simulink model "halfCar"  (R2017b)
settings: Solver=ode23t  StartTime=0.0  StopTime=10  FixedStep=0.05  RelTol=1e-3
settings Model: Creator=cs756  LastModifiedBy=cs756

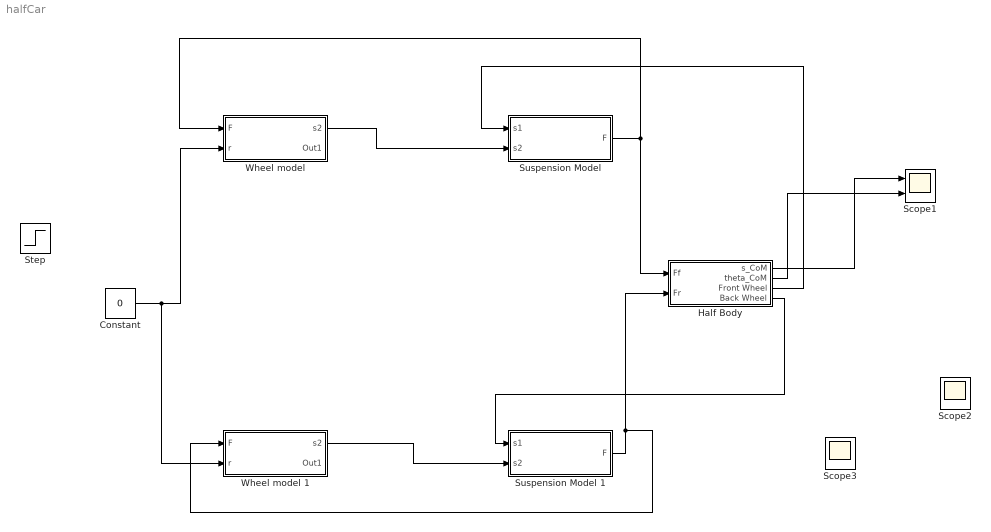
== system halfCar ==
  Constant : Constant  Value=0
  Half Body : Subsystem  mask{g=9.81, I=600, mb=500, a=1.25, b=1.4}
  Scope1 : Scope  NumInputPorts=2
  Scope2 : Scope
  Scope3 : Scope
  Step : Step  SampleTime=0
  "Suspension Model " : Subsystem  mask{cs1=1000, cs2=1000, ks=20000, ks2=20000, x0=2, x1=2}
      mask prompts: cs1 "Damper Compression coefficient"; cs2 "Damper Tension coefficient"; ks "Stiffness coefficient"; ks2 "Stiffness addition"; x0 "Elastic spring extension limit"; x1 "Damper motion range"
  Suspension Model 1 : Subsystem  mask{cs1=1000, cs2=1000, ks=20000, ks2=20000, x0=2, x1=2}
      mask prompts: cs1 "Damper Compression coefficient"; cs2 "Damper Tension coefficient"; ks "Stiffness coefficient"; ks2 "Stiffness addition"; x0 "Elastic spring extension limit"; x1 "Damper motion range"
  "Wheel model " : Subsystem  mask{kt=140000, kt2=140000, m2=20, g=9.81, x0=1}
      mask prompts: kt "Wheel soft stiffness"; kt2 "Wheel hard stiffness"; m2 "Wheel mass"; x0 "Wheel elastic extension limit"
  Wheel model 1 : Subsystem  mask{kt=140000, kt2=140000, m2=20, g=9.81, x0=1}
      mask prompts: kt "Wheel soft stiffness"; kt2 "Wheel hard stiffness"; m2 "Wheel mass"; x0 "Wheel elastic extension limit"
  wires:
  "Wheel model "/1(s2) -> "Suspension Model "/2(s2)
  Wheel model 1/1(s2) -> Suspension Model 1/2(s2)
  Constant/1 -> Wheel model 1/2(r), "Wheel model "/2(r)
  Half Body/4(Back Wheel) -> Suspension Model 1/1(s1)
  Half Body/3(Front Wheel) -> "Suspension Model "/1(s1)
  "Suspension Model "/1(F) -> Half Body/1(Ff), "Wheel model "/1(F)
  Suspension Model 1/1(F) -> Wheel model 1/1(F), Half Body/2(Fr)
  Half Body/1(s_CoM) -> Scope1/1
  Half Body/2(theta_CoM) -> Scope1/2

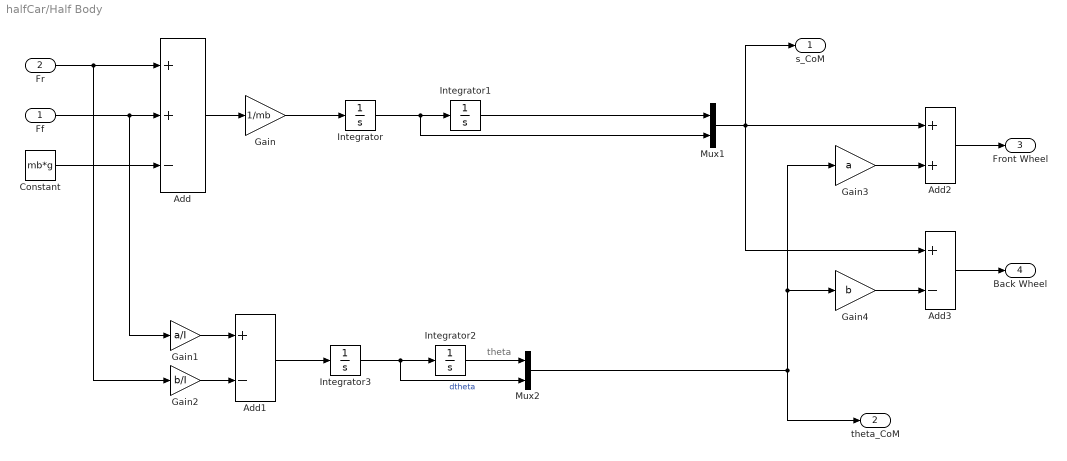
== system halfCar/Half Body ==
  note: theta
  Ff : Inport
  Fr : Inport  Port=2
  Add : Sum  Inputs=++-
  Add1 : Sum  Inputs=+-
  Add2 : Sum
  Add3 : Sum  Inputs=+-
  Constant : Constant  Value=mb*g
  Gain : Gain  Gain=1/mb
  Gain1 : Gain  Gain=a/I
  Gain2 : Gain  Gain=b/I
  Gain3 : Gain  Gain=a
  Gain4 : Gain  Gain=b
  Integrator{,1..3} (4 alike) : Integrator
  Mux1 : Mux  Inputs=2
  Mux2 : Mux  Inputs=2
  s_CoM : Outport
  theta_CoM : Outport  Port=2
  Front Wheel : Outport  Port=3
  Back Wheel : Outport  Port=4
  wires:
  Fr/1 -> Gain2/1, Add/1
  Constant/1 -> Add/3
  Add/1 -> Gain/1
  Gain/1 -> Integrator/1
  Integrator/1 -> Mux1/2, Integrator1/1
  Ff/1 -> Gain1/1, Add/2
  Gain2/1 -> Add1/2
  Gain1/1 -> Add1/1
  Integrator3/1 -> Mux2/2, Integrator2/1  "dtheta"
  Add1/1 -> Integrator3/1
  Integrator1/1 -> Mux1/1
  Integrator2/1 -> Mux2/1
  Gain3/1 -> Add2/2
  Gain4/1 -> Add3/2
  Add2/1 -> Front Wheel/1
  Add3/1 -> Back Wheel/1
  Mux2/1 -> Gain3/1, Gain4/1, theta_CoM/1
  Mux1/1 -> s_CoM/1, Add2/1, Add3/1

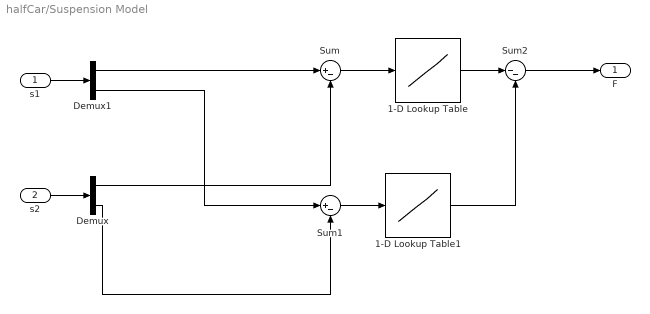
== system halfCar/Suspension Model  ==
  s1 : Inport
  s2 : Inport  Port=2
  1-D Lookup Table : Lookup_n-D  NumberOfTableDimensions=1  BreakpointsForDimension1=[-2*x0, -x0, x0, 2*x0]  Table=[-(ks+ks2)*x0,-ks*x0,ks*x0,(ks+ks2)*x0]  InternalRulePriority=Speed  RndMeth=Simplest  InputSameDT=on
  1-D Lookup Table1 : Lookup_n-D  NumberOfTableDimensions=1  BreakpointsForDimension1=[-x1, 0, x1]  Table=[-cs2*x1, 0, cs1*x1]  InternalRulePriority=Speed  RndMeth=Simplest  InputSameDT=on
  Demux : Demux  Outputs=2
  Demux1 : Demux  Outputs=2
  Sum : Sum  Inputs=|+-
  Sum1 : Sum  Inputs=|+-
  Sum2 : Sum  Inputs=|--
  F : Outport
  wires:
  Sum/1 -> 1-D Lookup Table/1
  Sum2/1 -> F/1
  s2/1 -> Demux/1
  Demux/1 -> Sum/2
  Demux/2 -> Sum1/2
  Demux1/1 -> Sum/1
  s1/1 -> Demux1/1
  Demux1/2 -> Sum1/1
  1-D Lookup Table/1 -> Sum2/1
  Sum1/1 -> 1-D Lookup Table1/1
  1-D Lookup Table1/1 -> Sum2/2

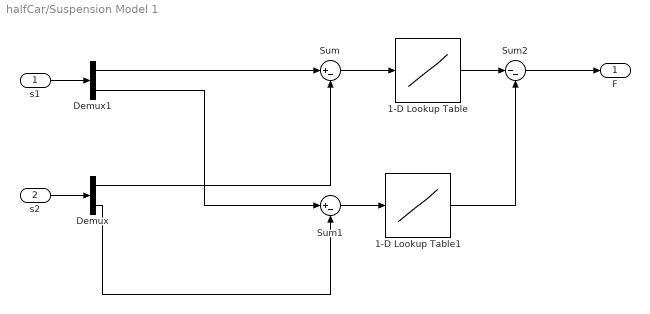
== system halfCar/Suspension Model 1 ==
  s1 : Inport
  s2 : Inport  Port=2
  1-D Lookup Table : Lookup_n-D  NumberOfTableDimensions=1  BreakpointsForDimension1=[-2*x0, -x0, x0, 2*x0]  Table=[-(ks+ks2)*x0,-ks*x0,ks*x0,(ks+ks2)*x0]  InternalRulePriority=Speed  RndMeth=Simplest  InputSameDT=on
  1-D Lookup Table1 : Lookup_n-D  NumberOfTableDimensions=1  BreakpointsForDimension1=[-x1, 0, x1]  Table=[-cs2*x1, 0, cs1*x1]  InternalRulePriority=Speed  RndMeth=Simplest  InputSameDT=on
  Demux : Demux  Outputs=2
  Demux1 : Demux  Outputs=2
  Sum : Sum  Inputs=|+-
  Sum1 : Sum  Inputs=|+-
  Sum2 : Sum  Inputs=|--
  F : Outport
  wires:
  Sum/1 -> 1-D Lookup Table/1
  Sum2/1 -> F/1
  s2/1 -> Demux/1
  Demux/1 -> Sum/2
  Demux/2 -> Sum1/2
  Demux1/1 -> Sum/1
  s1/1 -> Demux1/1
  Demux1/2 -> Sum1/1
  1-D Lookup Table/1 -> Sum2/1
  Sum1/1 -> 1-D Lookup Table1/1
  1-D Lookup Table1/1 -> Sum2/2

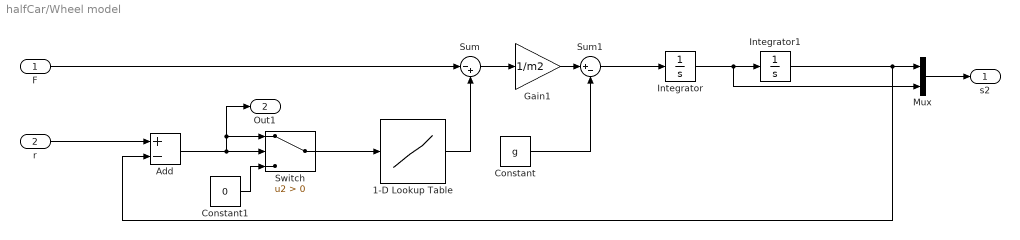
== system halfCar/Wheel model  ==
  F : Inport
  r : Inport  Port=2
  1-D Lookup Table : Lookup_n-D  NumberOfTableDimensions=1  BreakpointsForDimension1=[-2*x0, -x0, x0, 2*x0]  Table=[-(kt+kt2)*x0,-kt*x0,kt*x0,(kt+kt2)*x0]  InternalRulePriority=Speed  RndMeth=Simplest  InputSameDT=on
  Add : Sum  Inputs=+-
  Constant : Constant  Value=g
  Constant1 : Constant  Value=0
  Gain1 : Gain  Gain=1/m2
  Integrator : Integrator
  Integrator1 : Integrator
  Mux : Mux  Inputs=2
  Sum : Sum  Inputs=|-+
  Sum1 : Sum  Inputs=|+-
  Switch : Switch  Criteria=u2 > Threshold
  s2 : Outport
  Out1 : Outport  Port=2
  wires:
  r/1 -> Add/1
  F/1 -> Sum/1
  Add/1 -> Out1/1, Switch/1, Switch/2
  Constant1/1 -> Switch/3
  Switch/1 -> 1-D Lookup Table/1
  1-D Lookup Table/1 -> Sum/2
  Sum/1 -> Gain1/1
  Gain1/1 -> Sum1/1
  Constant/1 -> Sum1/2
  Sum1/1 -> Integrator/1
  Integrator/1 -> Mux/2, Integrator1/1
  Integrator1/1 -> Add/2, Mux/1
  Mux/1 -> s2/1

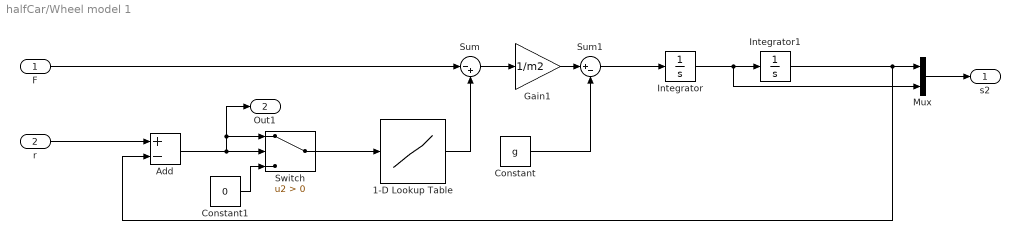
== system halfCar/Wheel model 1 ==
  F : Inport
  r : Inport  Port=2
  1-D Lookup Table : Lookup_n-D  NumberOfTableDimensions=1  BreakpointsForDimension1=[-2*x0, -x0, x0, 2*x0]  Table=[-(kt+kt2)*x0,-kt*x0,kt*x0,(kt+kt2)*x0]  InternalRulePriority=Speed  RndMeth=Simplest  InputSameDT=on
  Add : Sum  Inputs=+-
  Constant : Constant  Value=g
  Constant1 : Constant  Value=0
  Gain1 : Gain  Gain=1/m2
  Integrator : Integrator
  Integrator1 : Integrator
  Mux : Mux  Inputs=2
  Sum : Sum  Inputs=|-+
  Sum1 : Sum  Inputs=|+-
  Switch : Switch  Criteria=u2 > Threshold
  s2 : Outport
  Out1 : Outport  Port=2
  wires:
  r/1 -> Add/1
  F/1 -> Sum/1
  Add/1 -> Out1/1, Switch/1, Switch/2
  Constant1/1 -> Switch/3
  Switch/1 -> 1-D Lookup Table/1
  1-D Lookup Table/1 -> Sum/2
  Sum/1 -> Gain1/1
  Gain1/1 -> Sum1/1
  Constant/1 -> Sum1/2
  Sum1/1 -> Integrator/1
  Integrator/1 -> Mux/2, Integrator1/1
  Integrator1/1 -> Add/2, Mux/1
  Mux/1 -> s2/1
